simulink model "ragazzini_model"  (R2021b)
settings: Solver=ode4  StartTime=0.0  StopTime=30  FixedStep=1e-2  RelTol=1e-3
values from neighbouring files (symbols this model uses):
  k = 1    [ragazzini.m]
  k1 = 0.5    [ragazzini.m]
  k2 = 0.1    [ragazzini.m]
  tau = 0.5    [ragazzini.m]
settings Model: Creator=dmitr  LastModifiedBy=dmitr

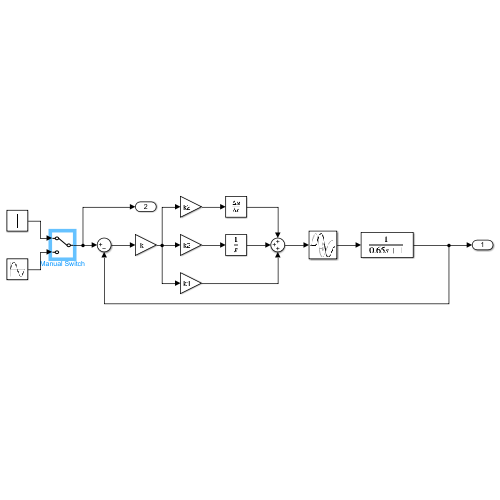
[thumbnail: Simulink's stored preview of the top-level diagram]
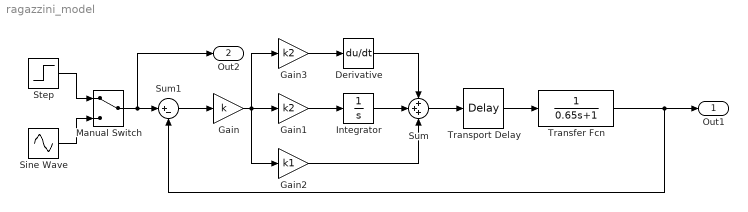
== system ragazzini_model ==
  Derivative : Derivative
  Gain : Gain  Gain=k
  Gain1 : Gain  Gain=k2
  Gain2 : Gain  Gain=k1
  Gain3 : Gain  Gain=k2
  Integrator : Integrator
  Manual Switch : ManualSwitch
  Sine Wave : Sin  SampleTime=0
  Step : Step  Time=0  SampleTime=0
  Sum : Sum  Inputs=+++
  Sum1 : Sum  Inputs=|+-
  Transfer Fcn : TransferFcn  Denominator=[0.65 1]
  Transport Delay : TransportDelay  DelayTime=tau
  Out1 : Outport
  Out2 : Outport  Port=2
  wires:
  Gain1/1 -> Integrator/1
  Gain3/1 -> Derivative/1
  Gain2/1 -> Sum/3
  Integrator/1 -> Sum/2
  Derivative/1 -> Sum/1
  Gain/1 -> Gain1/1, Gain3/1, Gain2/1
  Sum/1 -> Transport Delay/1
  Transport Delay/1 -> Transfer Fcn/1
  Sum1/1 -> Gain/1
  Step/1 -> Manual Switch/1
  Manual Switch/1 -> Out2/1, Sum1/1
  Sine Wave/1 -> Manual Switch/2
  Transfer Fcn/1 -> Sum1/2, Out1/1
